simulink model "Open_Loop_3DOF_Plant"  (R2024a)
settings: Solver=VariableStepAuto  StartTime=0.0  StopTime=5  RelTol=1e-3
model workspace: external: MATLAB File C:\Users\C27Derek.Weissinger\OneDrive - USAFA (AFAcademy.AF.edu)\Documents\Classes\Summer 26\Astro 499\Derek-Weissinger-GNC-Methods-2026\MATLAB + Simulink\vehicle_params.m (data not in the file)
values from neighbouring files (symbols this model uses):
  I = [1 0 0; 0 1 0; 0 0 1]    [dcm2euler.m]    (also in dcm2quat.m; euler2dcm.m; quat2dcm.m; vehicle_params.m = 0.048)
  Kd = 0.15    [vehicle_params.m]
  Ki = 0.01    [vehicle_params.m]
  Kp = 2    [vehicle_params.m]
  Lg = 0.28    [vehicle_params.m]
  m = 0.543    [vehicle_params.m]
  thetai = 5    [vehicle_params.m]
  Ts = 0.01    [vehicle_params.m]
libraries: aerolibutil x1, sharedutil x1, sharedtransform x1
settings Model: Creator=C28Derek.Weissinger  LastModifiedBy=C28Derek.Weissinger

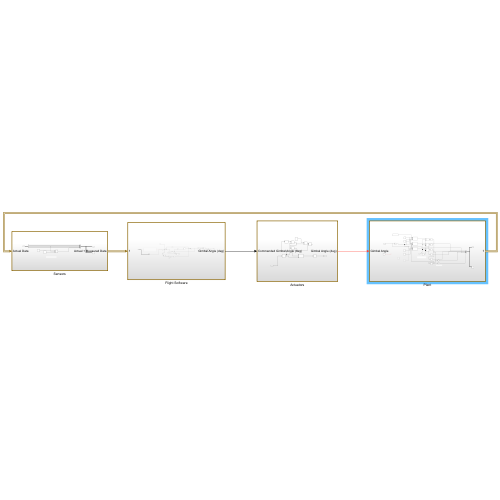
[thumbnail: Simulink's stored preview of the top-level diagram]
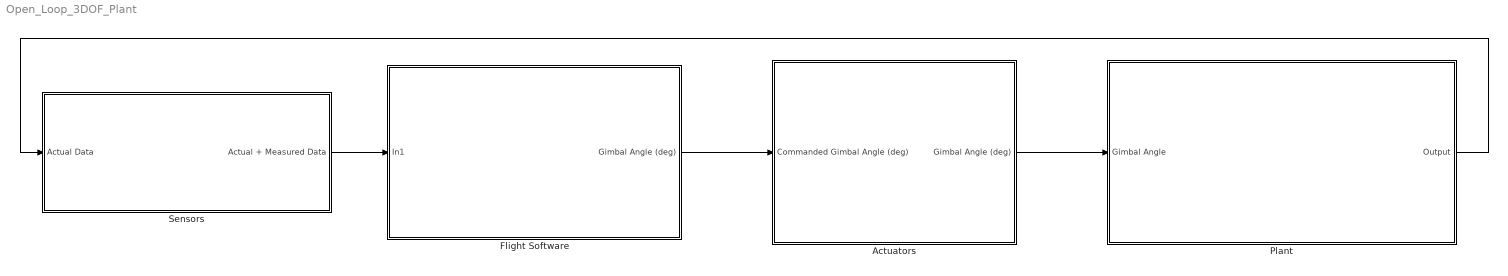
== system Open_Loop_3DOF_Plant ==
  Actuators : Subsystem
  Flight Software : Subsystem
  Plant : Subsystem
  Sensors : Subsystem
  wires:
  Plant/1(Output) -> Sensors/1(Actual Data)
  Sensors/1(Actual + Measured Data) -> Flight Software/1(In1)
  Flight Software/1(Gimbal Angle (deg)) -> Actuators/1(Commanded Gimbal Angle (deg))
  Actuators/1(Gimbal Angle (deg)) -> Plant/1(Gimbal Angle)

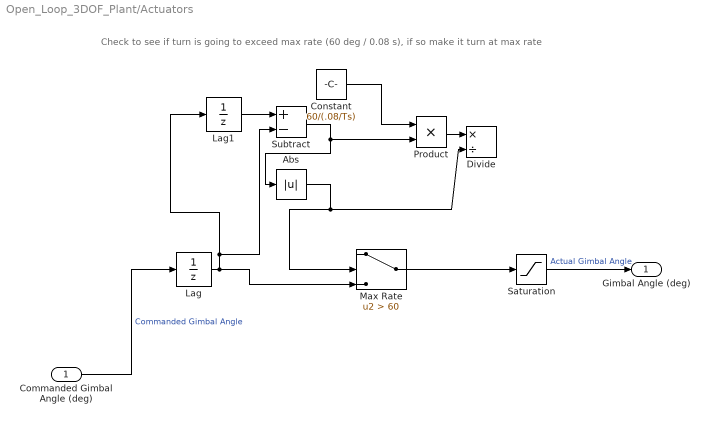
== system Open_Loop_3DOF_Plant/Actuators ==
  note: Check to see if turn is going to exceed max rate (60 deg / 0.08 s), if so make it turn at max rate
  Commanded Gimbal Angle (deg) : Inport
  Abs : Abs  SaturateOnIntegerOverflow=off
  Constant : Constant  Value=60/(.08/Ts)
  Divide : Product  Inputs=*/
  Lag : UnitDelay  SampleTime=Ts  HasFrameUpgradeWarning=on
  Lag1 : UnitDelay  SampleTime=0.08  HasFrameUpgradeWarning=on
  Max Rate : Switch  Criteria=u2 > Threshold  Threshold=60  SaturateOnIntegerOverflow=off  InputSameDT=off
  Product : Product
  Saturation : Saturate  UpperLimit=5  LowerLimit=-5
  Subtract : Sum  Inputs=+-
  Gimbal Angle (deg) : Outport
  wires:
  Commanded Gimbal Angle (deg)/1 -> Lag/1  "Commanded Gimbal Angle"
  Saturation/1 -> Gimbal Angle (deg)/1  "Actual Gimbal Angle"
  Lag/1 -> Max Rate/3, Subtract/2, Lag1/1
  Lag1/1 -> Subtract/1
  Subtract/1 -> Abs/1, Product/2
  Abs/1 -> Max Rate/2, Divide/2
  Constant/1 -> Product/1
  Product/1 -> Divide/1
  Max Rate/1 -> Saturation/1

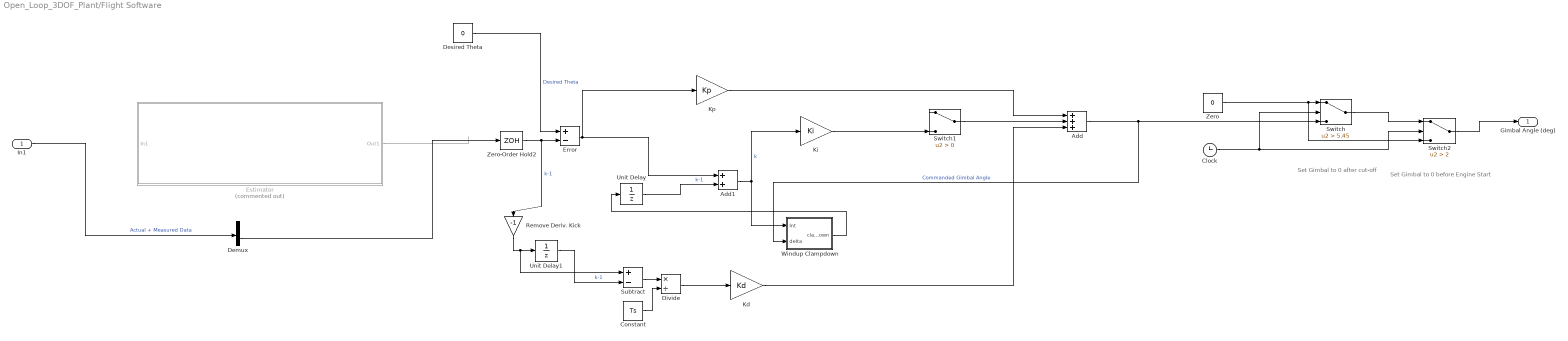
== system Open_Loop_3DOF_Plant/Flight Software ==
  note: Set Gimbal to 0 before Engine Start
  note: Set Gimbal to 0 after cut-off
  In1 : Inport
  Add : Sum  Inputs=+++
  Add1 : Sum
  Clock : Clock
  Constant : Constant  Value=Ts
  Demux : Demux  Outputs=8
  Desired Theta : Constant  Value=0
  Divide : Product  Inputs=*/
  Error : Sum  Inputs=+-
  Estimator : Subsystem  Commented=on
  Kd : Gain  Gain=Kd
  Ki : Gain  Gain=Ki
  Kp : Gain  Gain=Kp
  Remove Deriv. Kick : Gain  Gain=-1
  Subtract : Sum  Inputs=+-
  Switch : Switch  Criteria=u2 > Threshold  Threshold=5.45  SaturateOnIntegerOverflow=off  InputSameDT=off
  Switch1 : Switch  Criteria=u2 > Threshold  SaturateOnIntegerOverflow=off  InputSameDT=off
  Switch2 : Switch  Criteria=u2 > Threshold  Threshold=2  SaturateOnIntegerOverflow=off  InputSameDT=off
  Unit Delay : UnitDelay  SampleTime=Ts  HasFrameUpgradeWarning=on
  Unit Delay1 : UnitDelay  SampleTime=Ts  HasFrameUpgradeWarning=on
  Windup Clampdown : MATLAB Function  TreatAsAtomicUnit=on
  Zero : Constant  Value=0  OutDataTypeStr=Inherit: Inherit via back propagation
  Zero-Order Hold2 : ZeroOrderHold  SampleTime=Ts
  Gimbal Angle (deg) : Outport
  wires:
  In1/1 -> Demux/1  "Actual + Measured Data"
  Kp/1 -> Add/1
  Kd/1 -> Add/3
  Desired Theta/1 -> Error/1  "Desired Theta"
  Add/1 -> Windup Clampdown/2(delta), Switch/3  "Commanded Gimbal Angle"
  Unit Delay/1 -> Add1/2  "k-1"
  Add1/1 -> Windup Clampdown/1(Int), Ki/1  "k"
  Subtract/1 -> Divide/1
  Constant/1 -> Divide/2
  Divide/1 -> Kd/1
  Ki/1 -> Switch1/3
  Unit Delay1/1 -> Subtract/2  "k-1"
  Error/1 -> Kp/1, Add1/1
  Zero-Order Hold2/1 -> Error/2, Remove Deriv. Kick/1  "k-1"
  Clock/1 -> Switch2/2, Switch/2
  Zero/1 -> Switch2/3, Switch/1
  Switch/1 -> Switch2/1
  Switch1/1 -> Add/2
  Windup Clampdown/1(clampdown) -> Unit Delay/1
  Remove Deriv. Kick/1 -> Subtract/1, Unit Delay1/1
  Estimator/1(Out1) -> ?
  Switch2/1 -> Gimbal Angle (deg)/1
  Demux/6 -> Zero-Order Hold2/1

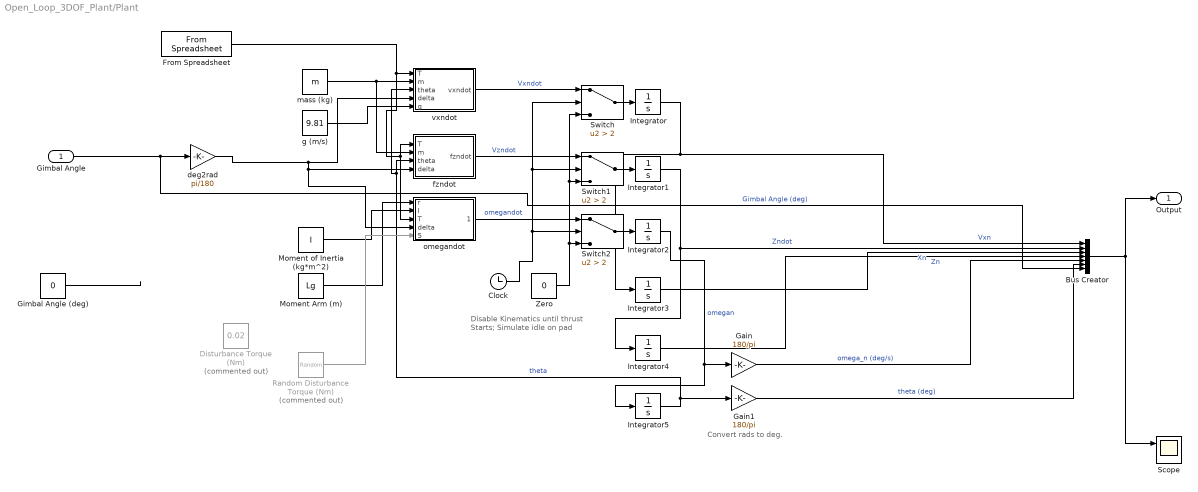
== system Open_Loop_3DOF_Plant/Plant ==
  note: Disable Kinematics until thrust
      | Starts; Simulate idle on pad
  note: Convert rads to deg.
  Gimbal Angle : Inport
  Bus Creator : BusCreator  Inputs=7
  Clock : Clock
  Disturbance Torque (Nm) : Constant  Commented=on  Value=0.02
  From Spreadsheet : FromSpreadsheet  FileName=Estes_F15.csv  SheetName=Estes_F15  ExtrapolationAfterLastDataPoint=Ground value
  Gain : Gain  Gain=180/pi
  Gain1 : Gain  Gain=180/pi
  Gimbal Angle (deg) : Constant  Value=0
  Integrator{,1..4} (5 alike) : Integrator
  Integrator5 : Integrator  InitialCondition=deg2rad(thetai)
  Moment Arm (m) : Constant  Value=Lg
  Moment of Inertia (kg*m^2) : Constant  Value=I
  Random Disturbance Torque (Nm) : RandomNumber  Commented=on  Mean=0.01  Variance=.02  SampleTime=0.1
  Scope : Scope  NumInputPorts=2
  Switch : Switch  Criteria=u2 > Threshold  Threshold=2  SaturateOnIntegerOverflow=off  InputSameDT=off
  Switch1 : Switch  Criteria=u2 > Threshold  Threshold=2  SaturateOnIntegerOverflow=off  InputSameDT=off
  Switch2 : Switch  Criteria=u2 > Threshold  Threshold=2  SaturateOnIntegerOverflow=off  InputSameDT=off
  Zero : Constant  Value=0  OutDataTypeStr=Inherit: Inherit via back propagation
  deg2rad : Gain  Gain=pi/180
  fzndot : MATLAB Function  TreatAsAtomicUnit=on
  g (m/s) : Constant  Value=9.81
  mass (kg) : Constant  Value=m
  omegandot : MATLAB Function  TreatAsAtomicUnit=on
  vxndot : MATLAB Function  TreatAsAtomicUnit=on
  Output : Outport
  wires:
  Integrator/1 -> Integrator3/1, Bus Creator/1  "Vxn"
  vxndot/1(vxndot) -> Switch/1  "Vxndot"
  fzndot/1(fzndot) -> Switch1/1  "Vzndot"
  Integrator2/1 -> Integrator5/1, Gain/1  "omegan"
  omegandot/1(omegandot) -> Switch2/1  "omegandot"
  Integrator3/1 -> Bus Creator/3  "Xn"
  Integrator1/1 -> Integrator4/1, Bus Creator/2  "Zndot"
  Integrator4/1 -> Bus Creator/4  "Zn"
  From Spreadsheet/1 -> omegandot/3(T), fzndot/1(T), vxndot/1(T)
  mass (kg)/1 -> fzndot/2(m), vxndot/2(m)
  g (m/s)/1 -> vxndot/5(g)
  Integrator5/1 -> Gain1/1, fzndot/3(theta), vxndot/3(theta)  "theta"
  Gimbal Angle (deg)/1 -> ?
  Moment Arm (m)/1 -> omegandot/1(r)
  Moment of Inertia (kg*m^2)/1 -> omegandot/2(I)
  Bus Creator/1 -> Output/1, Scope/1
  deg2rad/1 -> omegandot/4(delta), fzndot/4(delta), vxndot/4(delta)
  Gimbal Angle/1 -> Bus Creator/7, deg2rad/1  "Gimbal Angle (deg)"
  Gain/1 -> Bus Creator/5  "omega_n (deg/s)"
  Gain1/1 -> Bus Creator/6  "theta (deg)"
  Random Disturbance Torque (Nm)/1 -> omegandot/5(envtorque)
  Switch/1 -> Integrator/1
  Switch2/1 -> Integrator2/1
  Switch1/1 -> Integrator1/1
  Clock/1 -> Switch/2, Switch1/2, Switch2/2
  Zero/1 -> Switch/3, Switch1/3, Switch2/3

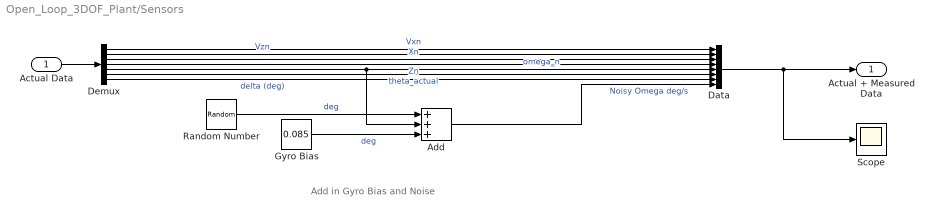
== system Open_Loop_3DOF_Plant/Sensors ==
  note: Add in Gyro Bias and Noise
  Actual Data : Inport
  Add : Sum  Inputs=+++
  Data : BusCreator  Inputs=8
  Demux : Demux  Outputs=7
  Gyro Bias : Constant  Value=0.085
  Random Number : RandomNumber  Mean=.25  SampleTime=0.01
  Scope : Scope
  Actual + Measured Data : Outport
  wires:
  Actual Data/1 -> Demux/1
  Demux/5 -> Add/2, Data/5  "omega_n"
  Random Number/1 -> Add/1  "deg"
  Gyro Bias/1 -> Add/3  "deg"
  Add/1 -> Data/8  "Noisy Omega deg/s"
  Demux/1 -> Data/1  "Vxn"
  Demux/2 -> Data/2  "Vzn"
  Demux/3 -> Data/3  "Xn"
  Demux/4 -> Data/4  "Zn"
  Demux/6 -> Data/6  "theta_actual"
  Data/1 -> Scope/1, Actual + Measured Data/1
  Demux/7 -> Data/7  "delta (deg)"

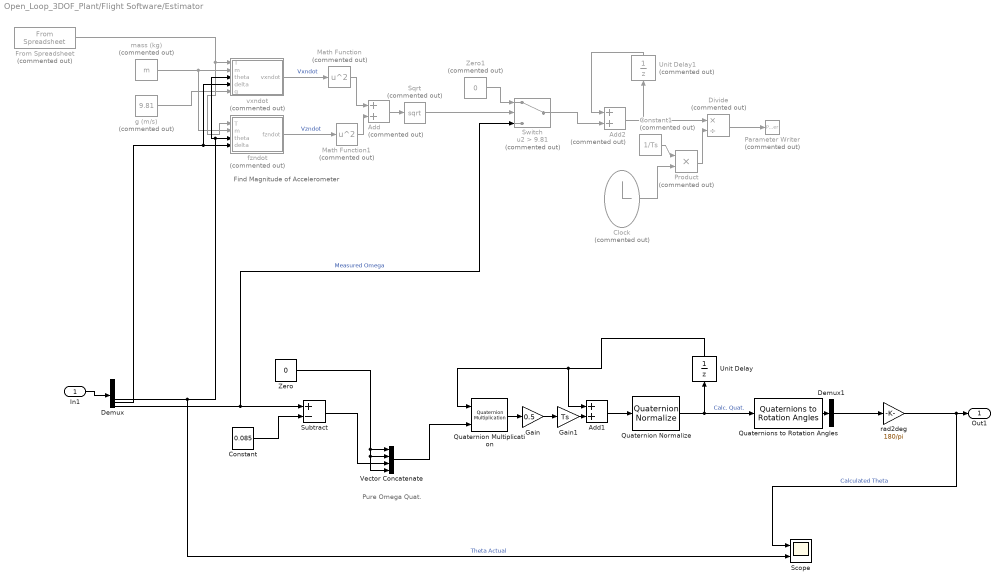
== system Open_Loop_3DOF_Plant/Flight Software/Estimator ==
  note: Find Magnitude of Accelerometer
  note: Pure Omega Quat.
  In1 : Inport
  Add : Sum  Commented=on
  Add1 : Sum
  Add2 : Sum  Commented=on
  Clock : Clock  Commented=on
  Constant : Constant  Value=0.085  SampleTime=-1
  Constant1 : Constant  Commented=on  Value=1/Ts
  Demux : Demux  Outputs=8
  Demux1 : Demux  Outputs=3
  Divide : Product  Commented=on  Inputs=*/
  From Spreadsheet : FromSpreadsheet  Commented=on  FileName=Estes_F15.csv  SheetName=Estes_F15  ExtrapolationAfterLastDataPoint=Ground value
  Gain : Gain  Gain=0.5
  Gain1 : Gain  Gain=Ts
  Math Function : Math  Commented=on  Operator=square
  Math Function1 : Math  Commented=on  Operator=square
  Parameter Writer : ParameterWriter  Commented=on  WorkspaceVariableName=MeasuredGyroBias  Destination=Base workspace variable
  Product : Product  Commented=on
  Quaternion Multiplication : aerolibutil/Quaternion Multiplication
  Quaternion Normalize : sharedutil/Quaternion Normalize  aMode=aMode
  Quaternions to Rotation Angles : sharedtransform/Quaternions to Rotation Angles  rotationOrder=ZYX  aMode=aMode
  Scope : Scope  NumInputPorts=2
  Sqrt : Sqrt  Commented=on
  Subtract : Sum  Inputs=+-
  Switch : Switch  Commented=on  Criteria=u2 > Threshold  Threshold=9.81  SaturateOnIntegerOverflow=off  InputSameDT=off
  Unit Delay : UnitDelay  InitialCondition=[1, 0, 0, 0]  SampleTime=Ts  HasFrameUpgradeWarning=on
  Unit Delay1 : UnitDelay  Commented=on  SampleTime=Ts  HasFrameUpgradeWarning=on
  Vector Concatenate : Concatenate  NumInputs=4
  Zero : Constant  Value=0  OutDataTypeStr=Inherit: Inherit via back propagation
  Zero1 : Constant  Commented=on  Value=0  OutDataTypeStr=Inherit: Inherit via back propagation
  fzndot : MATLAB Function  Commented=on  TreatAsAtomicUnit=on
  g (m/s) : Constant  Commented=on  Value=9.81
  mass (kg) : Constant  Commented=on  Value=m
  rad2deg : Gain  Gain=180/pi
  vxndot : MATLAB Function  Commented=on  TreatAsAtomicUnit=on
  Out1 : Outport
  wires:
  In1/1 -> Demux/1
  From Spreadsheet/1 -> fzndot/1(T), vxndot/1(T)
  mass (kg)/1 -> fzndot/2(m), vxndot/2(m)
  g (m/s)/1 -> vxndot/5(g)
  Demux/6 -> Scope/2, fzndot/3(theta), vxndot/3(theta)  "Theta Actual"
  Demux/7 -> fzndot/4(delta), vxndot/4(delta)
  vxndot/1(vxndot) -> Math Function/1  "Vxndot"
  fzndot/1(fzndot) -> Math Function1/1  "Vzndot"
  Math Function/1 -> Add/1
  Math Function1/1 -> Add/2
  Add/1 -> Sqrt/1
  Quaternions to Rotation Angles/1 -> Demux1/1
  Demux1/2 -> rad2deg/1
  rad2deg/1 -> Scope/1, Out1/1  "Calculated Theta"
  Unit Delay/1 -> Quaternion Multiplication/1, Add1/1
  Gain/1 -> Gain1/1
  Gain1/1 -> Add1/2
  Demux/8 -> Switch/3, Subtract/1  "Measured Omega"
  Zero/1 -> Vector Concatenate/4, Vector Concatenate/2, Vector Concatenate/1
  Quaternion Normalize/1 -> Quaternions to Rotation Angles/1, Unit Delay/1  "Calc. Quat."
  Add1/1 -> Quaternion Normalize/1
  Quaternion Multiplication/1 -> Gain/1
  Subtract/1 -> Vector Concatenate/3
  Constant/1 -> Subtract/2
  Vector Concatenate/1 -> Quaternion Multiplication/2
  Sqrt/1 -> Switch/2
  Zero1/1 -> Switch/1
  Switch/1 -> Add2/2
  Add2/1 -> Divide/1, Unit Delay1/1
  Unit Delay1/1 -> Add2/1
  Constant1/1 -> Product/1
  Clock/1 -> Product/2
  Product/1 -> Divide/2
  Divide/1 -> Parameter Writer/1

== matlab function Open_Loop_3DOF_Plant/Plant/fzndot ==
  data: T input; fzndot output; m input; theta input; delta input
function fzndot = fcn(T, m, theta, delta)
   fzndot = (T/m) * (sin(theta - delta));
end

== matlab function Open_Loop_3DOF_Plant/Plant/vxndot ==
  data: T input; vxndot output; m input; theta input; delta input; g input
function vxndot = fcn(T, m, theta, delta, g)
   vxndot = (T/m) * (cos(theta - delta)) - g;
end

== matlab function Open_Loop_3DOF_Plant/Plant/omegandot ==
  data: r input; omegandot output; I input; T input; delta input; envtorque input
function omegandot = fcn(r, I, T, delta, envtorque)

omegandot = (r/I) * T * delta + (envtorque/I);

end

== matlab function Open_Loop_3DOF_Plant/Flight Software/Windup Clampdown ==
  data: Int input; clampdown output; delta input
function clampdown = fcn(Int,delta)
if abs(Int) > 5 && Int*delta >0
        clampdown = 0;
else
    clampdown = Int;
end
end

== matlab function Open_Loop_3DOF_Plant/Flight Software/Estimator/fzndot ==
  data: T input; fzndot output; m input; theta input; delta input
function fzndot = fcn(T, m, theta, delta)
   fzndot = (T/m) * (sin(theta - delta));
end

== matlab function Open_Loop_3DOF_Plant/Flight Software/Estimator/vxndot ==
  data: T input; vxndot output; m input; theta input; delta input; g input
function vxndot = fcn(T, m, theta, delta, g)
   vxndot = (T/m) * (cos(theta - delta)) - g;
end
